simulink model "carrier_demod"  (Simulink 7.2)
settings: Solver=ode45  StartTime=0.0  StopTime=0.02  RelTol=1e-3
libraries: commsynccomp2 x2, dsparch4 x2, commfilt2 x1
settings Model: Creator=Administrator  LastModifiedBy=Administrator

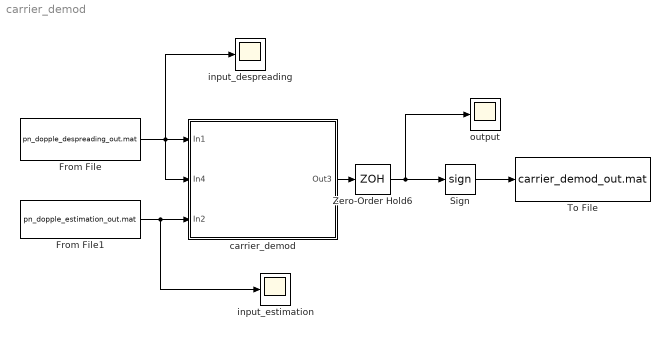
== system carrier_demod ==
  From File : FromFile  FileName=pn_dopple_despreading_out.mat  SampleTime=1/5.1e6
  From File1 : FromFile  FileName=pn_dopple_estimation_out.mat  SampleTime=1/5.1e6
  Sign : Signum
  To File : ToFile  Filename=carrier_demod_out.mat  MatrixName=ryuan
  Zero-Order Hold6 : ZeroOrderHold  SampleTime=1/1000
  carrier_demod : Subsystem
  input_despreading : Scope
      settings: YMin=1.45  YMax=1.825  SaveName=ScopeData7
  input_estimation : Scope
      settings: YMin=1.45  YMax=1.825  SaveName=ScopeData9
  output : Scope
      settings: YMin=1.45  YMax=1.825
  wires:
  carrier_demod/1(Out3) -> Zero-Order Hold6/1
  Zero-Order Hold6/1 -> Sign/1, output/1
  Sign/1 -> To File/1
  From File1/1 -> carrier_demod/3(In2), input_estimation/1
  From File/1 -> carrier_demod/2(In4), carrier_demod/1(In1), input_despreading/1

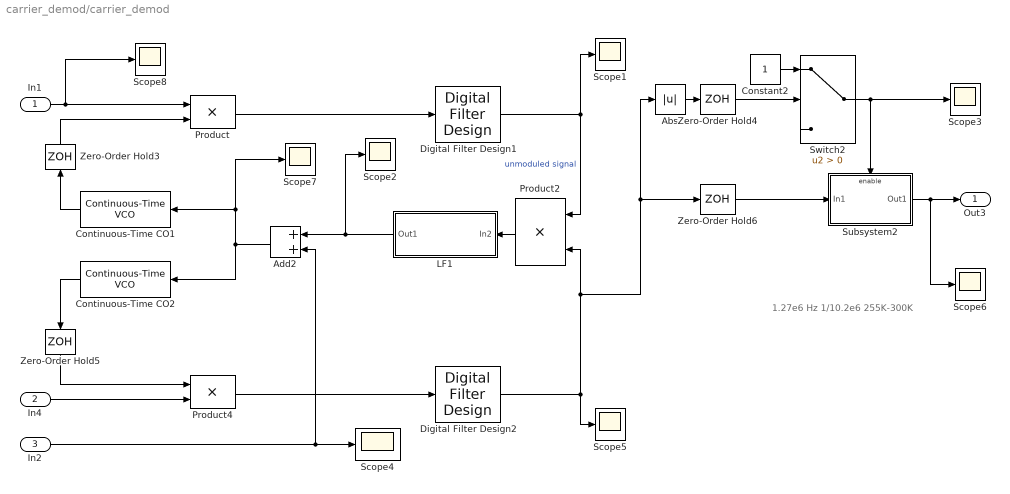
== system carrier_demod/carrier_demod ==
  note: 1.27e6 Hz
      |
      | 1/10.2e6
      |
      | 255K-300K
  In1 : Inport  OutDataType=sfix(16)  OutScaling=2^0
  In4 : Inport  Port=2  OutDataType=sfix(16)  OutScaling=2^0
  In2 : Inport  Port=3  OutDataType=sfix(16)  OutScaling=2^0
  Abs : Abs
  Add2 : Sum  Orientation=left  OutDataType=sfix(16)  OutScaling=2^-10
  Constant2 : Constant  OutDataType=sfix(16)  OutScaling=2^0
  Continuous-Time CO1 : commsynccomp2/Continuous-Time VCO  Orientation=left  SystemSampleTime=-1  Ac=2  Fc=5.0e5  Kc=100  Ph=pi/2
  Continuous-Time CO2 : commsynccomp2/Continuous-Time VCO  Orientation=left  SystemSampleTime=-1  Ac=2  Fc=5.0e5  Kc=100  Ph=0
  Digital Filter Design1 : dsparch4/Digital Filter Design  SystemSampleTime=-1  mwdsp_browser_bugfix_var=off
  Digital Filter Design2 : dsparch4/Digital Filter Design  SystemSampleTime=-1  mwdsp_browser_bugfix_var=off
  LF1 : Subsystem  Orientation=left
  Product : Product  OutDataType=sfix(16)  OutScaling=2^0  SaturateOnIntegerOverflow=on  OutDataTypeStr=Inherit: Same as first input
  Product2 : Product  Orientation=left  OutDataType=sfix(16)  OutScaling=2^0  SaturateOnIntegerOverflow=on  OutDataTypeStr=Inherit: Same as first input
  Product4 : Product  OutDataType=sfix(16)  OutScaling=2^0  SaturateOnIntegerOverflow=on  OutDataTypeStr=Inherit: Same as first input
  Scope{1..8} (8 alike) : Scope
      Scope1 settings: TimeRange=0.06427185951473757  YMin=-2  YMax=2  MaxDataPoints=100000
      Scope2 settings: TimeRange=0.03  YMin=-1.5  YMax=1.75  SaveName=ScopeData6  MaxDataPoints=100000
      Scope3 settings: YMin=-2  YMax=2  SaveName=ScopeData35
      Scope4 settings: TimeRange=0.06427185951473757  YMin=-200  YMax=200  SaveName=ScopeData8  MaxDataPoints=100000
      Scope5 settings: TimeRange=0.06427185951473757  YMin=-2  YMax=2  SaveName=ScopeData2  MaxDataPoints=100000
      Scope6 settings: YMin=-2  YMax=2  SaveName=ScopeData3
      Scope7 settings: TimeRange=0.06427185951473757  YMin=113000  YMax=129000  SaveName=ScopeData4  MaxDataPoints=100000
      Scope8 settings: TimeRange=0.06427185951473757  YMin=-2  YMax=2  SaveName=ScopeData5  MaxDataPoints=100000
  Subsystem2 : Subsystem  TreatAsAtomicUnit=on
  Switch2 : Switch  Criteria=u2 > Threshold
  Zero-Order Hold3 : ZeroOrderHold  Orientation=up  SampleTime=1/5.1e6
  Zero-Order Hold4 : ZeroOrderHold  SampleTime=1/1e5
  Zero-Order Hold5 : ZeroOrderHold  Orientation=down  SampleTime=1/5.1e6
  Zero-Order Hold6 : ZeroOrderHold  SampleTime=1/5.1e6
  Out3 : Outport  OutDataType=sfix(16)  OutScaling=2^0
  wires:
  In2/1 -> Scope4/1, Add2/2
  Add2/1 -> Scope7/1, Continuous-Time CO1/1, Continuous-Time CO2/1
  Zero-Order Hold5/1 -> Product4/1
  In4/1 -> Product4/2
  Product4/1 -> Digital Filter Design2/1
  Continuous-Time CO2/1 -> Zero-Order Hold5/1
  Digital Filter Design2/1 -> Scope5/1, Product2/2, Zero-Order Hold6/1, Abs/1
  Zero-Order Hold6/1 -> Subsystem2/1(In1)
  Abs/1 -> Zero-Order Hold4/1
  Switch2/1 -> Subsystem2/Enable, Scope3/1
  Zero-Order Hold4/1 -> Switch2/2
  Constant2/1 -> Switch2/1
  Subsystem2/1(Out1) -> Scope6/1, Out3/1
  Zero-Order Hold3/1 -> Product/2
  LF1/1(Out1) -> Add2/1, Scope2/1
  In1/1 -> Scope8/1, Product/1
  Digital Filter Design1/1 -> Scope1/1, Product2/1  "unmoduled signal"
  Continuous-Time CO1/1 -> Zero-Order Hold3/1
  Product/1 -> Digital Filter Design1/1
  Product2/1 -> LF1/1(In2)

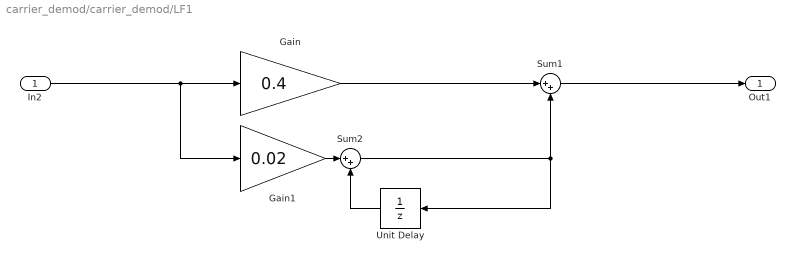
== system carrier_demod/carrier_demod/LF1 ==
  In2 : Inport  OutDataType=sfix(16)  OutScaling=2^0
  Gain : Gain  Gain=0.4  ParameterDataType=sfix(16)  ParameterScaling=2^0  OutDataType=sfix(16)  OutScaling=2^0  SaturateOnIntegerOverflow=on  OutDataTypeStr=Inherit: Same as input  ParamDataTypeStr=Inherit: Same as input
  Gain1 : Gain  Gain=0.02  ParameterDataType=sfix(16)  ParameterScaling=2^0  OutDataType=sfix(16)  OutScaling=2^0  SaturateOnIntegerOverflow=on  OutDataTypeStr=Inherit: Same as input  ParamDataTypeStr=Inherit: Same as input
  Sum1 : Sum  Inputs=|++  OutDataType=sfix(16)  OutScaling=2^0  SaturateOnIntegerOverflow=on  InputSameDT=on  OutDataTypeStr=Inherit: Same as first input
  Sum2 : Sum  Inputs=|++  OutDataType=sfix(16)  OutScaling=2^0  SaturateOnIntegerOverflow=on  InputSameDT=on  OutDataTypeStr=Inherit: Same as first input
  Unit Delay : UnitDelay  Orientation=left  SampleTime=1/1e5
  Out1 : Outport  OutDataType=sfix(16)  OutScaling=2^0
  wires:
  Sum2/1 -> Unit Delay/1, Sum1/2
  Sum1/1 -> Out1/1
  Gain/1 -> Sum1/1
  Unit Delay/1 -> Sum2/2
  Gain1/1 -> Sum2/1
  In2/1 -> Gain/1, Gain1/1

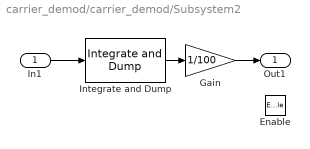
== system carrier_demod/carrier_demod/Subsystem2 ==
  In1 : Inport  OutDataType=sfix(16)  OutScaling=2^0
  Enable : EnablePort
  Gain : Gain  Gain=1/100  ParameterDataType=sfix(16)  ParameterScaling=2^0  OutDataType=sfix(16)  OutScaling=2^0
  Integrate and Dump : commfilt2/Integrate and Dump  DialogController=commDDGCreate  DialogControllerArgs=DataTag2  obssamples=100  offsetsamples=0  nodump=off  roundingMode=Floor  overflowMode=off
  Out1 : Outport  OutDataType=sfix(16)  OutScaling=2^0
  wires:
  Gain/1 -> Out1/1
  In1/1 -> Integrate and Dump/1
  Integrate and Dump/1 -> Gain/1
